simulink library "carnotUIBK"  (R2024b)
settings: Solver=VariableStepAuto  StartTime=0.0  StopTime=10.0  RelTol=1e-3  EnableMultiTasking=on
values from neighbouring files (symbols this model uses):
  area = area + room(kk).area    [THERMALZONE.m]
  boundary = BOUNDARY()    [BUILDING.m]
  building = obj    [BUILDING.m]
  C = zeros(1,length(d)+1)    [CONSTRUCTION.m]
  cp = str2num(value)    [CONSTRUCTION.m]
  pos = find(d_layer>0)    [CONSTRUCTION.m]
  rho = str2num(value)    [CONSTRUCTION.m]
  type = 1    [CONSTRUCTION.m]
  zone = obj.zone(ind)    [THERMALZONE.m]
undefined symbols (not defined in the file or in its folder): A, amb_factor, B, const, control, Dd, get_building, height, p, Qdot_C, Qdot_H, Qdot_I_electricity, Qdot_I_light, Qdot_I_person, Qdot_S, Qdot_T_ground, Qdot_T_neighbour, Qdot_T_opaque, Qdot_T_window, Qdot_V_infiltration, Qdot_V_mech, Qdot_V_window, r_frame, solar_ratio, solar_ratio1, solar_ratio2, Tc, Tr, Ts, Uvalue, view_factor, wall, wallsurface, window, window_height, window_heigth, window_width, windowsurface, x_CO2, x_H2O, x_VOC, z
libraries: carnot x105, $bdroot x22, simulink x18, simulink_extras x14
(part 6 of 13)

== system carnotUIBK/HVAC/HVAC_2001_ventilation system simple/ventilation_zone 6 ==
  note: ASSUMPTION: mdot_air_in = mdot_air_out !
  note: AIR VENTILATION outdoors - indoors
  note: x_sup = x_amb + (x_ext - x_amb) * eta_x
  AIB : Inport
  WDB : Inport  Port=2
  Vdot : Inport  Port=3
  Enable : EnablePort
  "\"air\"" : Constant  Value=2
  "1/h -> 1/s" : Gain  Gain=1/3600  SaturateOnIntegerOverflow=on  OutDataTypeStr=Inherit: Same as input  ParamDataTypeStr=Inherit: Same as input
  Bus Creator1 : BusCreator  Inputs=2
  Bus Selector : BusSelector  OutputSignals=Temperature_Ambient,Relative_Humidity,Station_Pressure
  Bus Selector1 : BusSelector  OutputSignals=Tc,x_H2O,x_CO2
  Constant : Constant  Value=zeros(1,2)
  Constant1 : Constant  Value=zeros(1,5)
  Constant2 : Constant  Value=zeros(1,7)
  Constant3 : Constant  Value=1-eta
  Constant4 : Constant  Value=0
  Constant5 : Constant  Value=eta_x
  Density : carnot/Basic/Material_Properties/Density  VariantControl=CarlibClassic  INPUTARGUMENTS=state variables (classic)  DEBUGLEVEL=NOLEVEL  MAXTOTALWARNINGS=inf  MAXCONSECUTIVEWARNINGS=inf  WRITETOFILE=0  FILENAME='errors.txt'
      settings: SourceProductName=Carnot
  Fcn : Fcn  Expr=u / (1+u)
  Fcn1 : Fcn  Expr=u / (1+u)
  Integrator : Integrator
  Mux1 : Mux  Inputs=[1 1]
  Mux3 : Mux  Inputs=[1 2 1 1 1 5 1 7]
  Mux4 : Mux  Inputs=2
  Product1 : Product  InputSameDT=on  SaturateOnIntegerOverflow=on  OutDataTypeStr=Inherit: Same as first input
  Product2 : Product  InputSameDT=on  SaturateOnIntegerOverflow=on  OutDataTypeStr=Inherit: Same as first input
  Product3 : Product  InputSameDT=on  SaturateOnIntegerOverflow=on  OutDataTypeStr=Inherit: Same as first input
  Product4 : Product  Inputs=4  InputSameDT=on  SaturateOnIntegerOverflow=on  OutDataTypeStr=Inherit: Same as first input
  RelHum2x : carnot/Basic/Material_Properties/RelHum2x
      settings: SourceProductName=Carnot
  Subsystem : Subsystem
  Sum : Sum  Inputs=-+  InputSameDT=on  SaturateOnIntegerOverflow=on  OutDataTypeStr=Inherit: Same as first input
  Sum1 : Sum  Inputs=-+  InputSameDT=on  SaturateOnIntegerOverflow=on  OutDataTypeStr=Inherit: Same as first input
  Sum2 : Sum  Inputs=++-  InputSameDT=on  SaturateOnIntegerOverflow=on  OutDataTypeStr=Inherit: Same as first input
  Terminator : Terminator
  cp Constant : Constant  Value=1006.8
  rho(CO2) / rho(air) * CO2norm (kg/kg) : Constant  Value=1.529*CO2norm
  "[S]" : Outport  VectorParamsAs1DForOutWhenUnconnected=off
  "[HVAC]" : Outport  Port=2  VectorParamsAs1DForOutWhenUnconnected=off
  wires:
  Fcn1/1 -> Sum2/1, Sum1/1
  Fcn/1 -> Sum1/2, Sum2/3
  Product2/1 -> Mux3/4  "mdot_H2O"
  Sum2/1 -> Product2/2  "x_sup"
  Product1/1 -> Sum2/2
  Sum1/1 -> Product1/2
  Constant5/1 -> Product1/1
  Subsystem/1(mdot_H2O) -> Terminator/1  "mdot_H2O"
  Constant4/1 -> Mux3/3
  Vdot/1 -> "1/h -> 1/s"/1
  Mux3/1 -> "[S]"/1
  Subsystem/2(mdot_CO2) -> Mux3/5  "mdot_CO2"
  WDB/1 -> Bus Selector/1
  AIB/1 -> Bus Selector1/1
  Density/1 -> Product3/2
  Bus Selector/3 -> RelHum2x/2, Density/2  "<Station_Pressure>"
  Bus Selector/2 -> RelHum2x/3  "<Relative_Humidity>"
  Bus Selector/1 -> RelHum2x/1, Density/1, Sum/2  "<Temperature_Ambient>"
  RelHum2x/1 -> Density/4, Mux4/1, Fcn1/1  "x_H2O"
  "\"air\""/1 -> Density/3
  Mux1/1 -> Subsystem/2(x_in)  "[x_H2O, x_CO2]_in"
  Bus Selector1/1 -> Sum/1  "<Tc>"
  Mux4/1 -> Subsystem/3(x_out)
  rho(CO2) / rho(air) * CO2norm (kg/kg)/1 -> Mux4/2  "x_CO2"
  Sum/1 -> Product4/2  "dT"
  cp Constant/1 -> Product4/3  "cp"
  Product3/1 -> Product4/4, Product2/1, Subsystem/1(mdot_air)
  Bus Selector1/2 -> Mux1/1, Fcn/1  "<x_H2O>"
  Bus Selector1/3 -> Mux1/2  "<x_CO2>"
  Constant/1 -> Mux3/2
  Constant1/1 -> Mux3/6
  Constant2/1 -> Mux3/8
  Constant3/1 -> Product4/1
  "1/h -> 1/s"/1 -> Product3/1
  Bus Creator1/1 -> "[HVAC]"/1
  Product4/1 -> Mux3/7, Integrator/1, Bus Creator1/1, Mux3/1  "ventilation power"
  Integrator/1 -> Bus Creator1/2  "ventilation energy"

== system carnotUIBK/HVAC/HVAC_2001_ventilation system simple/ventilation_zone 7 ==
  note: ASSUMPTION: mdot_air_in = mdot_air_out !
  note: AIR VENTILATION outdoors - indoors
  note: x_sup = x_amb + (x_ext - x_amb) * eta_x
  AIB : Inport
  WDB : Inport  Port=2
  Vdot : Inport  Port=3
  Enable : EnablePort
  "\"air\"" : Constant  Value=2
  "1/h -> 1/s" : Gain  Gain=1/3600  SaturateOnIntegerOverflow=on  OutDataTypeStr=Inherit: Same as input  ParamDataTypeStr=Inherit: Same as input
  Bus Creator1 : BusCreator  Inputs=2
  Bus Selector : BusSelector  OutputSignals=Temperature_Ambient,Relative_Humidity,Station_Pressure
  Bus Selector1 : BusSelector  OutputSignals=Tc,x_H2O,x_CO2
  Constant : Constant  Value=zeros(1,2)
  Constant1 : Constant  Value=zeros(1,5)
  Constant2 : Constant  Value=zeros(1,7)
  Constant3 : Constant  Value=1-eta
  Constant4 : Constant  Value=0
  Constant5 : Constant  Value=eta_x
  Density : carnot/Basic/Material_Properties/Density  VariantControl=CarlibClassic  INPUTARGUMENTS=state variables (classic)  DEBUGLEVEL=NOLEVEL  MAXTOTALWARNINGS=inf  MAXCONSECUTIVEWARNINGS=inf  WRITETOFILE=0  FILENAME='errors.txt'
      settings: SourceProductName=Carnot
  Fcn : Fcn  Expr=u / (1+u)
  Fcn1 : Fcn  Expr=u / (1+u)
  Integrator : Integrator
  Mux1 : Mux  Inputs=[1 1]
  Mux3 : Mux  Inputs=[1 2 1 1 1 5 1 7]
  Mux4 : Mux  Inputs=2
  Product1 : Product  InputSameDT=on  SaturateOnIntegerOverflow=on  OutDataTypeStr=Inherit: Same as first input
  Product2 : Product  InputSameDT=on  SaturateOnIntegerOverflow=on  OutDataTypeStr=Inherit: Same as first input
  Product3 : Product  InputSameDT=on  SaturateOnIntegerOverflow=on  OutDataTypeStr=Inherit: Same as first input
  Product4 : Product  Inputs=4  InputSameDT=on  SaturateOnIntegerOverflow=on  OutDataTypeStr=Inherit: Same as first input
  RelHum2x : carnot/Basic/Material_Properties/RelHum2x
      settings: SourceProductName=Carnot
  Subsystem : Subsystem
  Sum : Sum  Inputs=-+  InputSameDT=on  SaturateOnIntegerOverflow=on  OutDataTypeStr=Inherit: Same as first input
  Sum1 : Sum  Inputs=-+  InputSameDT=on  SaturateOnIntegerOverflow=on  OutDataTypeStr=Inherit: Same as first input
  Sum2 : Sum  Inputs=++-  InputSameDT=on  SaturateOnIntegerOverflow=on  OutDataTypeStr=Inherit: Same as first input
  Terminator : Terminator
  cp Constant : Constant  Value=1006.8
  rho(CO2) / rho(air) * CO2norm (kg/kg) : Constant  Value=1.529*CO2norm
  "[S]" : Outport  VectorParamsAs1DForOutWhenUnconnected=off
  "[HVAC]" : Outport  Port=2  VectorParamsAs1DForOutWhenUnconnected=off
  wires:
  Fcn1/1 -> Sum2/1, Sum1/1
  Fcn/1 -> Sum1/2, Sum2/3
  Product2/1 -> Mux3/4  "mdot_H2O"
  Sum2/1 -> Product2/2  "x_sup"
  Product1/1 -> Sum2/2
  Sum1/1 -> Product1/2
  Constant5/1 -> Product1/1
  Subsystem/1(mdot_H2O) -> Terminator/1  "mdot_H2O"
  Constant4/1 -> Mux3/3
  Vdot/1 -> "1/h -> 1/s"/1
  Mux3/1 -> "[S]"/1
  Subsystem/2(mdot_CO2) -> Mux3/5  "mdot_CO2"
  WDB/1 -> Bus Selector/1
  AIB/1 -> Bus Selector1/1
  Density/1 -> Product3/2
  Bus Selector/3 -> RelHum2x/2, Density/2  "<Station_Pressure>"
  Bus Selector/2 -> RelHum2x/3  "<Relative_Humidity>"
  Bus Selector/1 -> RelHum2x/1, Density/1, Sum/2  "<Temperature_Ambient>"
  RelHum2x/1 -> Density/4, Mux4/1, Fcn1/1  "x_H2O"
  "\"air\""/1 -> Density/3
  Mux1/1 -> Subsystem/2(x_in)  "[x_H2O, x_CO2]_in"
  Bus Selector1/1 -> Sum/1  "<Tc>"
  Mux4/1 -> Subsystem/3(x_out)
  rho(CO2) / rho(air) * CO2norm (kg/kg)/1 -> Mux4/2  "x_CO2"
  Sum/1 -> Product4/2  "dT"
  cp Constant/1 -> Product4/3  "cp"
  Product3/1 -> Product4/4, Product2/1, Subsystem/1(mdot_air)
  Bus Selector1/2 -> Mux1/1, Fcn/1  "<x_H2O>"
  Bus Selector1/3 -> Mux1/2  "<x_CO2>"
  Constant/1 -> Mux3/2
  Constant1/1 -> Mux3/6
  Constant2/1 -> Mux3/8
  Constant3/1 -> Product4/1
  "1/h -> 1/s"/1 -> Product3/1
  Bus Creator1/1 -> "[HVAC]"/1
  Product4/1 -> Mux3/7, Integrator/1, Bus Creator1/1, Mux3/1  "ventilation power"
  Integrator/1 -> Bus Creator1/2  "ventilation energy"

== system carnotUIBK/HVAC/HVAC_2001_ventilation system simple/ventilation_zone 8 ==
  note: ASSUMPTION: mdot_air_in = mdot_air_out !
  note: AIR VENTILATION outdoors - indoors
  note: x_sup = x_amb + (x_ext - x_amb) * eta_x
  AIB : Inport
  WDB : Inport  Port=2
  Vdot : Inport  Port=3
  Enable : EnablePort
  "\"air\"" : Constant  Value=2
  "1/h -> 1/s" : Gain  Gain=1/3600  SaturateOnIntegerOverflow=on  OutDataTypeStr=Inherit: Same as input  ParamDataTypeStr=Inherit: Same as input
  Bus Creator1 : BusCreator  Inputs=2
  Bus Selector : BusSelector  OutputSignals=Temperature_Ambient,Relative_Humidity,Station_Pressure
  Bus Selector1 : BusSelector  OutputSignals=Tc,x_H2O,x_CO2
  Constant : Constant  Value=zeros(1,2)
  Constant1 : Constant  Value=zeros(1,5)
  Constant2 : Constant  Value=zeros(1,7)
  Constant3 : Constant  Value=1-eta
  Constant4 : Constant  Value=0
  Constant5 : Constant  Value=eta_x
  Density : carnot/Basic/Material_Properties/Density  VariantControl=CarlibClassic  INPUTARGUMENTS=state variables (classic)  DEBUGLEVEL=NOLEVEL  MAXTOTALWARNINGS=inf  MAXCONSECUTIVEWARNINGS=inf  WRITETOFILE=0  FILENAME='errors.txt'
      settings: SourceProductName=Carnot
  Fcn : Fcn  Expr=u / (1+u)
  Fcn1 : Fcn  Expr=u / (1+u)
  Integrator : Integrator
  Mux1 : Mux  Inputs=[1 1]
  Mux3 : Mux  Inputs=[1 2 1 1 1 5 1 7]
  Mux4 : Mux  Inputs=2
  Product1 : Product  InputSameDT=on  SaturateOnIntegerOverflow=on  OutDataTypeStr=Inherit: Same as first input
  Product2 : Product  InputSameDT=on  SaturateOnIntegerOverflow=on  OutDataTypeStr=Inherit: Same as first input
  Product3 : Product  InputSameDT=on  SaturateOnIntegerOverflow=on  OutDataTypeStr=Inherit: Same as first input
  Product4 : Product  Inputs=4  InputSameDT=on  SaturateOnIntegerOverflow=on  OutDataTypeStr=Inherit: Same as first input
  RelHum2x : carnot/Basic/Material_Properties/RelHum2x
      settings: SourceProductName=Carnot
  Subsystem : Subsystem
  Sum : Sum  Inputs=-+  InputSameDT=on  SaturateOnIntegerOverflow=on  OutDataTypeStr=Inherit: Same as first input
  Sum1 : Sum  Inputs=-+  InputSameDT=on  SaturateOnIntegerOverflow=on  OutDataTypeStr=Inherit: Same as first input
  Sum2 : Sum  Inputs=++-  InputSameDT=on  SaturateOnIntegerOverflow=on  OutDataTypeStr=Inherit: Same as first input
  Terminator : Terminator
  cp Constant : Constant  Value=1006.8
  rho(CO2) / rho(air) * CO2norm (kg/kg) : Constant  Value=1.529*CO2norm
  "[S]" : Outport  VectorParamsAs1DForOutWhenUnconnected=off
  "[HVAC]" : Outport  Port=2  VectorParamsAs1DForOutWhenUnconnected=off
  wires:
  Fcn1/1 -> Sum2/1, Sum1/1
  Fcn/1 -> Sum1/2, Sum2/3
  Product2/1 -> Mux3/4  "mdot_H2O"
  Sum2/1 -> Product2/2  "x_sup"
  Product1/1 -> Sum2/2
  Sum1/1 -> Product1/2
  Constant5/1 -> Product1/1
  Subsystem/1(mdot_H2O) -> Terminator/1  "mdot_H2O"
  Constant4/1 -> Mux3/3
  Vdot/1 -> "1/h -> 1/s"/1
  Mux3/1 -> "[S]"/1
  Subsystem/2(mdot_CO2) -> Mux3/5  "mdot_CO2"
  WDB/1 -> Bus Selector/1
  AIB/1 -> Bus Selector1/1
  Density/1 -> Product3/2
  Bus Selector/3 -> RelHum2x/2, Density/2  "<Station_Pressure>"
  Bus Selector/2 -> RelHum2x/3  "<Relative_Humidity>"
  Bus Selector/1 -> RelHum2x/1, Density/1, Sum/2  "<Temperature_Ambient>"
  RelHum2x/1 -> Density/4, Mux4/1, Fcn1/1  "x_H2O"
  "\"air\""/1 -> Density/3
  Mux1/1 -> Subsystem/2(x_in)  "[x_H2O, x_CO2]_in"
  Bus Selector1/1 -> Sum/1  "<Tc>"
  Mux4/1 -> Subsystem/3(x_out)
  rho(CO2) / rho(air) * CO2norm (kg/kg)/1 -> Mux4/2  "x_CO2"
  Sum/1 -> Product4/2  "dT"
  cp Constant/1 -> Product4/3  "cp"
  Product3/1 -> Product4/4, Product2/1, Subsystem/1(mdot_air)
  Bus Selector1/2 -> Mux1/1, Fcn/1  "<x_H2O>"
  Bus Selector1/3 -> Mux1/2  "<x_CO2>"
  Constant/1 -> Mux3/2
  Constant1/1 -> Mux3/6
  Constant2/1 -> Mux3/8
  Constant3/1 -> Product4/1
  "1/h -> 1/s"/1 -> Product3/1
  Bus Creator1/1 -> "[HVAC]"/1
  Product4/1 -> Mux3/7, Integrator/1, Bus Creator1/1, Mux3/1  "ventilation power"
  Integrator/1 -> Bus Creator1/2  "ventilation energy"

== system carnotUIBK/HVAC/HVAC_2001_ventilation system simple/ventilation_zone 9 ==
  note: ASSUMPTION: mdot_air_in = mdot_air_out !
  note: AIR VENTILATION outdoors - indoors
  note: x_sup = x_amb + (x_ext - x_amb) * eta_x
  AIB : Inport
  WDB : Inport  Port=2
  Vdot : Inport  Port=3
  Enable : EnablePort
  "\"air\"" : Constant  Value=2
  "1/h -> 1/s" : Gain  Gain=1/3600  SaturateOnIntegerOverflow=on  OutDataTypeStr=Inherit: Same as input  ParamDataTypeStr=Inherit: Same as input
  Bus Creator1 : BusCreator  Inputs=2
  Bus Selector : BusSelector  OutputSignals=Temperature_Ambient,Relative_Humidity,Station_Pressure
  Bus Selector1 : BusSelector  OutputSignals=Tc,x_H2O,x_CO2
  Constant : Constant  Value=zeros(1,2)
  Constant1 : Constant  Value=zeros(1,5)
  Constant2 : Constant  Value=zeros(1,7)
  Constant3 : Constant  Value=1-eta
  Constant4 : Constant  Value=0
  Constant5 : Constant  Value=eta_x
  Density : carnot/Basic/Material_Properties/Density  VariantControl=CarlibClassic  INPUTARGUMENTS=state variables (classic)  DEBUGLEVEL=NOLEVEL  MAXTOTALWARNINGS=inf  MAXCONSECUTIVEWARNINGS=inf  WRITETOFILE=0  FILENAME='errors.txt'
      settings: SourceProductName=Carnot
  Fcn : Fcn  Expr=u / (1+u)
  Fcn1 : Fcn  Expr=u / (1+u)
  Integrator : Integrator
  Mux1 : Mux  Inputs=[1 1]
  Mux3 : Mux  Inputs=[1 2 1 1 1 5 1 7]
  Mux4 : Mux  Inputs=2
  Product1 : Product  InputSameDT=on  SaturateOnIntegerOverflow=on  OutDataTypeStr=Inherit: Same as first input
  Product2 : Product  InputSameDT=on  SaturateOnIntegerOverflow=on  OutDataTypeStr=Inherit: Same as first input
  Product3 : Product  InputSameDT=on  SaturateOnIntegerOverflow=on  OutDataTypeStr=Inherit: Same as first input
  Product4 : Product  Inputs=4  InputSameDT=on  SaturateOnIntegerOverflow=on  OutDataTypeStr=Inherit: Same as first input
  RelHum2x : carnot/Basic/Material_Properties/RelHum2x
      settings: SourceProductName=Carnot
  Subsystem : Subsystem
  Sum : Sum  Inputs=-+  InputSameDT=on  SaturateOnIntegerOverflow=on  OutDataTypeStr=Inherit: Same as first input
  Sum1 : Sum  Inputs=-+  InputSameDT=on  SaturateOnIntegerOverflow=on  OutDataTypeStr=Inherit: Same as first input
  Sum2 : Sum  Inputs=++-  InputSameDT=on  SaturateOnIntegerOverflow=on  OutDataTypeStr=Inherit: Same as first input
  Terminator : Terminator
  cp Constant : Constant  Value=1006.8
  rho(CO2) / rho(air) * CO2norm (kg/kg) : Constant  Value=1.529*CO2norm
  "[S]" : Outport  VectorParamsAs1DForOutWhenUnconnected=off
  "[HVAC]" : Outport  Port=2  VectorParamsAs1DForOutWhenUnconnected=off
  wires:
  Fcn1/1 -> Sum2/1, Sum1/1
  Fcn/1 -> Sum1/2, Sum2/3
  Product2/1 -> Mux3/4  "mdot_H2O"
  Sum2/1 -> Product2/2  "x_sup"
  Product1/1 -> Sum2/2
  Sum1/1 -> Product1/2
  Constant5/1 -> Product1/1
  Subsystem/1(mdot_H2O) -> Terminator/1  "mdot_H2O"
  Constant4/1 -> Mux3/3
  Vdot/1 -> "1/h -> 1/s"/1
  Mux3/1 -> "[S]"/1
  Subsystem/2(mdot_CO2) -> Mux3/5  "mdot_CO2"
  WDB/1 -> Bus Selector/1
  AIB/1 -> Bus Selector1/1
  Density/1 -> Product3/2
  Bus Selector/3 -> RelHum2x/2, Density/2  "<Station_Pressure>"
  Bus Selector/2 -> RelHum2x/3  "<Relative_Humidity>"
  Bus Selector/1 -> RelHum2x/1, Density/1, Sum/2  "<Temperature_Ambient>"
  RelHum2x/1 -> Density/4, Mux4/1, Fcn1/1  "x_H2O"
  "\"air\""/1 -> Density/3
  Mux1/1 -> Subsystem/2(x_in)  "[x_H2O, x_CO2]_in"
  Bus Selector1/1 -> Sum/1  "<Tc>"
  Mux4/1 -> Subsystem/3(x_out)
  rho(CO2) / rho(air) * CO2norm (kg/kg)/1 -> Mux4/2  "x_CO2"
  Sum/1 -> Product4/2  "dT"
  cp Constant/1 -> Product4/3  "cp"
  Product3/1 -> Product4/4, Product2/1, Subsystem/1(mdot_air)
  Bus Selector1/2 -> Mux1/1, Fcn/1  "<x_H2O>"
  Bus Selector1/3 -> Mux1/2  "<x_CO2>"
  Constant/1 -> Mux3/2
  Constant1/1 -> Mux3/6
  Constant2/1 -> Mux3/8
  Constant3/1 -> Product4/1
  "1/h -> 1/s"/1 -> Product3/1
  Bus Creator1/1 -> "[HVAC]"/1
  Product4/1 -> Mux3/7, Integrator/1, Bus Creator1/1, Mux3/1  "ventilation power"
  Integrator/1 -> Bus Creator1/2  "ventilation energy"

== system carnotUIBK/HVAC/HVAC_9001_window shading/Transfer Fcn (with initial states) ==
  In1 : Inport
  State Space : StateSpace  A=A  B=B  C=C  D=Dd  InitialCondition=X0
  Out1 : Outport  InitialOutput=0  VectorParamsAs1DForOutWhenUnconnected=off
  wires:
  In1/1 -> State Space/1
  State Space/1 -> Out1/1

== system carnotUIBK/HVAC/HVAC_9002_window opening/window opening 1 ==
  setpoint : Inport
  AIB : Inport  Port=2
  WDB : Inport  Port=3
  Enable : EnablePort
  Add : Sum
  Bus Selector1 : BusSelector  OutputSignals=Temperature_Ambient
  Bus Selector5 : BusSelector  OutputSignals=Ts,Tc,p,x_H2O
  Product : Product
  Saturation : Saturate  UpperLimit=1  LowerLimit=0
  Sum : Sum  Inputs=|-+
  Sum1 : Sum  Inputs=|+-
  Sum2 : Sum  Inputs=|-+
  Transfer Fcn (with initial states) : Subsystem  mask(Transfer Function with Initial States){N=[1], D=[600 1], X0=0}
      mask prompts: N "Numerator:"; D "Denominator:"; X0 "Initial conditions:"
      mask help: Vector expressions for numerator, and denominator. Coefficients are in descending powers of s.
      mask init:
      | [A,B,C,Dd]=tf2ss(N,D);if (isempty(X0));[m,n]=size(A);X0=zeros(1,m); end;
      mask Help: Specify the initial states for the transfer function.  The state ordering is determined by the m-file tf2ss.  There is no unique mapping of the states in a transfer function to states in a state-space representation.  However, tf2ss will consistently use the same mapping for a given transfer function.
      mask Display: dpoly(N,D,'s')
  Transfer Fcn (with initial states)1 : Subsystem  mask(Transfer Function with Initial States){N=[1], D=[600 1], X0=0}
      mask prompts: N "Numerator:"; D "Denominator:"; X0 "Initial conditions:"
      mask help: Vector expressions for numerator, and denominator. Coefficients are in descending powers of s.
      mask init:
      | [A,B,C,Dd]=tf2ss(N,D);if (isempty(X0));[m,n]=size(A);X0=zeros(1,m); end;
      mask Help: Specify the initial states for the transfer function.  The state ordering is determined by the m-file tf2ss.  There is no unique mapping of the states in a transfer function to states in a state-space representation.  However, tf2ss will consistently use the same mapping for a given transfer function.
      mask Display: dpoly(N,D,'s')
  Transfer Fcn (with initial states)2 : Subsystem  mask(Transfer Function with Initial States){N=[1], D=[600 1], X0=0}
      mask prompts: N "Numerator:"; D "Denominator:"; X0 "Initial conditions:"
      mask help: Vector expressions for numerator, and denominator. Coefficients are in descending powers of s.
      mask init:
      | [A,B,C,Dd]=tf2ss(N,D);if (isempty(X0));[m,n]=size(A);X0=zeros(1,m); end;
      mask Help: Specify the initial states for the transfer function.  The state ordering is determined by the m-file tf2ss.  There is no unique mapping of the states in a transfer function to states in a state-space representation.  However, tf2ss will consistently use the same mapping for a given transfer function.
      mask Display: dpoly(N,D,'s')
  on/off ambient : Relay  OnSwitchValue=0.5  OffSwitchValue=-0.5
  on/off hum : Relay  OnSwitchValue=0.5  OffSwitchValue=-0.5
  on/off roomtemp : Relay  OnSwitchValue=0.5  OffSwitchValue=-0.5
  setpoint humidity : Constant  Value=85
  x2RelHum_UIBK : carnot/Basic/Material_Properties/x2RelHum
      settings: SourceProductName=Carnot
  state : Outport  VectorParamsAs1DForOutWhenUnconnected=off
  wires:
  AIB/1 -> Bus Selector5/1
  setpoint/1 -> Sum/1
  Bus Selector5/1 -> Transfer Fcn (with initial states)/1(In1)  "<Ts>"
  Sum/1 -> on/off roomtemp/1
  on/off roomtemp/1 -> Product/1
  WDB/1 -> Bus Selector1/1
  Bus Selector1/1 -> Transfer Fcn (with initial states)2/1(In1)  "<Temperature_Ambient>"
  Sum1/1 -> on/off ambient/1
  on/off ambient/1 -> Product/2
  Bus Selector5/2 -> x2RelHum_UIBK/1  "<Tc>"
  Bus Selector5/3 -> x2RelHum_UIBK/2  "<p>"
  Bus Selector5/4 -> x2RelHum_UIBK/3  "<x_H2O>"
  Sum2/1 -> on/off hum/1
  x2RelHum_UIBK/1 -> Transfer Fcn (with initial states)1/1(In1)
  setpoint humidity/1 -> Sum2/1
  Add/1 -> Saturation/1
  Product/1 -> Add/2
  on/off hum/1 -> Add/1
  Saturation/1 -> state/1
  Transfer Fcn (with initial states)/1(Out1) -> Sum1/1, Sum/2
  Transfer Fcn (with initial states)2/1(Out1) -> Sum1/2
  Transfer Fcn (with initial states)1/1(Out1) -> Sum2/2

== system carnotUIBK/HVAC/HVAC_9002_window opening/window opening 2 ==
  setpoint : Inport
  AIB : Inport  Port=2
  WDB : Inport  Port=3
  Enable : EnablePort
  Add : Sum
  Bus Selector1 : BusSelector  OutputSignals=Temperature_Ambient
  Bus Selector5 : BusSelector  OutputSignals=Ts,Tc,p,x_H2O
  Product : Product
  Saturation : Saturate  UpperLimit=1  LowerLimit=0
  Sum : Sum  Inputs=|-+
  Sum1 : Sum  Inputs=|+-
  Sum2 : Sum  Inputs=|-+
  Transfer Fcn (with initial states)1 : Subsystem  mask(Transfer Function with Initial States){N=[1], D=[600 1], X0=0}
      mask prompts: N "Numerator:"; D "Denominator:"; X0 "Initial conditions:"
      mask help: Vector expressions for numerator, and denominator. Coefficients are in descending powers of s.
      mask init:
      | [A,B,C,Dd]=tf2ss(N,D);if (isempty(X0));[m,n]=size(A);X0=zeros(1,m); end;
      mask Help: Specify the initial states for the transfer function.  The state ordering is determined by the m-file tf2ss.  There is no unique mapping of the states in a transfer function to states in a state-space representation.  However, tf2ss will consistently use the same mapping for a given transfer function.
      mask Display: dpoly(N,D,'s')
  Transfer Fcn (with initial states)2 : Subsystem  mask(Transfer Function with Initial States){N=[1], D=[600 1], X0=0}
      mask prompts: N "Numerator:"; D "Denominator:"; X0 "Initial conditions:"
      mask help: Vector expressions for numerator, and denominator. Coefficients are in descending powers of s.
      mask init:
      | [A,B,C,Dd]=tf2ss(N,D);if (isempty(X0));[m,n]=size(A);X0=zeros(1,m); end;
      mask Help: Specify the initial states for the transfer function.  The state ordering is determined by the m-file tf2ss.  There is no unique mapping of the states in a transfer function to states in a state-space representation.  However, tf2ss will consistently use the same mapping for a given transfer function.
      mask Display: dpoly(N,D,'s')
  Transfer Fcn (with initial states)3 : Subsystem  mask(Transfer Function with Initial States){N=[1], D=[600 1], X0=0}
      mask prompts: N "Numerator:"; D "Denominator:"; X0 "Initial conditions:"
      mask help: Vector expressions for numerator, and denominator. Coefficients are in descending powers of s.
      mask init:
      | [A,B,C,Dd]=tf2ss(N,D);if (isempty(X0));[m,n]=size(A);X0=zeros(1,m); end;
      mask Help: Specify the initial states for the transfer function.  The state ordering is determined by the m-file tf2ss.  There is no unique mapping of the states in a transfer function to states in a state-space representation.  However, tf2ss will consistently use the same mapping for a given transfer function.
      mask Display: dpoly(N,D,'s')
  on/off ambient : Relay  OnSwitchValue=0.5  OffSwitchValue=-0.5
  on/off hum : Relay  OnSwitchValue=0.5  OffSwitchValue=-0.5
  on/off roomtemp : Relay  OnSwitchValue=0.5  OffSwitchValue=-0.5
  setpoint humidity : Constant  Value=85
  x2RelHum_UIBK : carnot/Basic/Material_Properties/x2RelHum
      settings: SourceProductName=Carnot
  state : Outport  VectorParamsAs1DForOutWhenUnconnected=off
  wires:
  Transfer Fcn (with initial states)1/1(Out1) -> Sum2/2
  Transfer Fcn (with initial states)3/1(Out1) -> Sum1/2
  Transfer Fcn (with initial states)2/1(Out1) -> Sum/2, Sum1/1
  Saturation/1 -> state/1
  on/off hum/1 -> Add/1
  Product/1 -> Add/2
  Add/1 -> Saturation/1
  setpoint humidity/1 -> Sum2/1
  x2RelHum_UIBK/1 -> Transfer Fcn (with initial states)1/1(In1)
  Sum2/1 -> on/off hum/1
  Bus Selector5/4 -> x2RelHum_UIBK/3  "<x_H2O>"
  Bus Selector5/3 -> x2RelHum_UIBK/2  "<p>"
  Bus Selector5/2 -> x2RelHum_UIBK/1  "<Tc>"
  on/off ambient/1 -> Product/2
  Sum1/1 -> on/off ambient/1
  Bus Selector1/1 -> Transfer Fcn (with initial states)3/1(In1)  "<Temperature_Ambient>"
  WDB/1 -> Bus Selector1/1
  on/off roomtemp/1 -> Product/1
  Sum/1 -> on/off roomtemp/1
  Bus Selector5/1 -> Transfer Fcn (with initial states)2/1(In1)  "<Ts>"
  setpoint/1 -> Sum/1
  AIB/1 -> Bus Selector5/1

== system carnotUIBK/HVAC/HVAC_9002_window opening/window opening 3 ==
  setpoint : Inport
  AIB : Inport  Port=2
  WDB : Inport  Port=3
  Enable : EnablePort
  Add : Sum
  Bus Selector1 : BusSelector  OutputSignals=Temperature_Ambient
  Bus Selector5 : BusSelector  OutputSignals=Ts,Tc,p,x_H2O
  Product : Product
  Saturation : Saturate  UpperLimit=1  LowerLimit=0
  Sum : Sum  Inputs=|-+
  Sum1 : Sum  Inputs=|+-
  Sum2 : Sum  Inputs=|-+
  Transfer Fcn (with initial states)1 : Subsystem  mask(Transfer Function with Initial States){N=[1], D=[600 1], X0=0}
      mask prompts: N "Numerator:"; D "Denominator:"; X0 "Initial conditions:"
      mask help: Vector expressions for numerator, and denominator. Coefficients are in descending powers of s.
      mask init:
      | [A,B,C,Dd]=tf2ss(N,D);if (isempty(X0));[m,n]=size(A);X0=zeros(1,m); end;
      mask Help: Specify the initial states for the transfer function.  The state ordering is determined by the m-file tf2ss.  There is no unique mapping of the states in a transfer function to states in a state-space representation.  However, tf2ss will consistently use the same mapping for a given transfer function.
      mask Display: dpoly(N,D,'s')
  Transfer Fcn (with initial states)2 : Subsystem  mask(Transfer Function with Initial States){N=[1], D=[600 1], X0=0}
      mask prompts: N "Numerator:"; D "Denominator:"; X0 "Initial conditions:"
      mask help: Vector expressions for numerator, and denominator. Coefficients are in descending powers of s.
      mask init:
      | [A,B,C,Dd]=tf2ss(N,D);if (isempty(X0));[m,n]=size(A);X0=zeros(1,m); end;
      mask Help: Specify the initial states for the transfer function.  The state ordering is determined by the m-file tf2ss.  There is no unique mapping of the states in a transfer function to states in a state-space representation.  However, tf2ss will consistently use the same mapping for a given transfer function.
      mask Display: dpoly(N,D,'s')
  Transfer Fcn (with initial states)3 : Subsystem  mask(Transfer Function with Initial States){N=[1], D=[600 1], X0=0}
      mask prompts: N "Numerator:"; D "Denominator:"; X0 "Initial conditions:"
      mask help: Vector expressions for numerator, and denominator. Coefficients are in descending powers of s.
      mask init:
      | [A,B,C,Dd]=tf2ss(N,D);if (isempty(X0));[m,n]=size(A);X0=zeros(1,m); end;
      mask Help: Specify the initial states for the transfer function.  The state ordering is determined by the m-file tf2ss.  There is no unique mapping of the states in a transfer function to states in a state-space representation.  However, tf2ss will consistently use the same mapping for a given transfer function.
      mask Display: dpoly(N,D,'s')
  on/off ambient : Relay  OnSwitchValue=0.5  OffSwitchValue=-0.5
  on/off hum : Relay  OnSwitchValue=0.5  OffSwitchValue=-0.5
  on/off roomtemp : Relay  OnSwitchValue=0.5  OffSwitchValue=-0.5
  setpoint humidity : Constant  Value=85
  x2RelHum_UIBK : carnot/Basic/Material_Properties/x2RelHum
      settings: SourceProductName=Carnot
  state : Outport  VectorParamsAs1DForOutWhenUnconnected=off
  wires:
  AIB/1 -> Bus Selector5/1
  setpoint/1 -> Sum/1
  Bus Selector5/1 -> Transfer Fcn (with initial states)3/1(In1)  "<Ts>"
  Sum/1 -> on/off roomtemp/1
  on/off roomtemp/1 -> Product/1
  WDB/1 -> Bus Selector1/1
  Bus Selector1/1 -> Transfer Fcn (with initial states)2/1(In1)  "<Temperature_Ambient>"
  Sum1/1 -> on/off ambient/1
  on/off ambient/1 -> Product/2
  Bus Selector5/2 -> x2RelHum_UIBK/1  "<Tc>"
  Bus Selector5/3 -> x2RelHum_UIBK/2  "<p>"
  Bus Selector5/4 -> x2RelHum_UIBK/3  "<x_H2O>"
  Sum2/1 -> on/off hum/1
  x2RelHum_UIBK/1 -> Transfer Fcn (with initial states)1/1(In1)
  setpoint humidity/1 -> Sum2/1
  Add/1 -> Saturation/1
  Product/1 -> Add/2
  on/off hum/1 -> Add/1
  Saturation/1 -> state/1
  Transfer Fcn (with initial states)3/1(Out1) -> Sum1/1, Sum/2
  Transfer Fcn (with initial states)2/1(Out1) -> Sum1/2
  Transfer Fcn (with initial states)1/1(Out1) -> Sum2/2

== system carnotUIBK/HVAC/HVAC_9002_window opening/window opening 4 ==
  setpoint : Inport
  AIB : Inport  Port=2
  WDB : Inport  Port=3
  Enable : EnablePort
  Add : Sum
  Bus Selector1 : BusSelector  OutputSignals=Temperature_Ambient
  Bus Selector5 : BusSelector  OutputSignals=Ts,Tc,p,x_H2O
  Product : Product
  Saturation : Saturate  UpperLimit=1  LowerLimit=0
  Sum : Sum  Inputs=|-+
  Sum1 : Sum  Inputs=|+-
  Sum2 : Sum  Inputs=|-+
  Transfer Fcn (with initial states)1 : Subsystem  mask(Transfer Function with Initial States){N=[1], D=[600 1], X0=0}
      mask prompts: N "Numerator:"; D "Denominator:"; X0 "Initial conditions:"
      mask help: Vector expressions for numerator, and denominator. Coefficients are in descending powers of s.
      mask init:
      | [A,B,C,Dd]=tf2ss(N,D);if (isempty(X0));[m,n]=size(A);X0=zeros(1,m); end;
      mask Help: Specify the initial states for the transfer function.  The state ordering is determined by the m-file tf2ss.  There is no unique mapping of the states in a transfer function to states in a state-space representation.  However, tf2ss will consistently use the same mapping for a given transfer function.
      mask Display: dpoly(N,D,'s')
  Transfer Fcn (with initial states)2 : Subsystem  mask(Transfer Function with Initial States){N=[1], D=[600 1], X0=0}
      mask prompts: N "Numerator:"; D "Denominator:"; X0 "Initial conditions:"
      mask help: Vector expressions for numerator, and denominator. Coefficients are in descending powers of s.
      mask init:
      | [A,B,C,Dd]=tf2ss(N,D);if (isempty(X0));[m,n]=size(A);X0=zeros(1,m); end;
      mask Help: Specify the initial states for the transfer function.  The state ordering is determined by the m-file tf2ss.  There is no unique mapping of the states in a transfer function to states in a state-space representation.  However, tf2ss will consistently use the same mapping for a given transfer function.
      mask Display: dpoly(N,D,'s')
  Transfer Fcn (with initial states)3 : Subsystem  mask(Transfer Function with Initial States){N=[1], D=[600 1], X0=0}
      mask prompts: N "Numerator:"; D "Denominator:"; X0 "Initial conditions:"
      mask help: Vector expressions for numerator, and denominator. Coefficients are in descending powers of s.
      mask init:
      | [A,B,C,Dd]=tf2ss(N,D);if (isempty(X0));[m,n]=size(A);X0=zeros(1,m); end;
      mask Help: Specify the initial states for the transfer function.  The state ordering is determined by the m-file tf2ss.  There is no unique mapping of the states in a transfer function to states in a state-space representation.  However, tf2ss will consistently use the same mapping for a given transfer function.
      mask Display: dpoly(N,D,'s')
  on/off ambient : Relay  OnSwitchValue=0.5  OffSwitchValue=-0.5
  on/off hum : Relay  OnSwitchValue=0.5  OffSwitchValue=-0.5
  on/off roomtemp : Relay  OnSwitchValue=0.5  OffSwitchValue=-0.5
  setpoint humidity : Constant  Value=85
  x2RelHum_UIBK : carnot/Basic/Material_Properties/x2RelHum
      settings: SourceProductName=Carnot
  state : Outport  VectorParamsAs1DForOutWhenUnconnected=off
  wires:
  Transfer Fcn (with initial states)1/1(Out1) -> Sum2/2
  Transfer Fcn (with initial states)2/1(Out1) -> Sum1/2
  Transfer Fcn (with initial states)3/1(Out1) -> Sum/2, Sum1/1
  Saturation/1 -> state/1
  on/off hum/1 -> Add/1
  Product/1 -> Add/2
  Add/1 -> Saturation/1
  setpoint humidity/1 -> Sum2/1
  x2RelHum_UIBK/1 -> Transfer Fcn (with initial states)1/1(In1)
  Sum2/1 -> on/off hum/1
  Bus Selector5/4 -> x2RelHum_UIBK/3  "<x_H2O>"
  Bus Selector5/3 -> x2RelHum_UIBK/2  "<p>"
  Bus Selector5/2 -> x2RelHum_UIBK/1  "<Tc>"
  on/off ambient/1 -> Product/2
  Sum1/1 -> on/off ambient/1
  Bus Selector1/1 -> Transfer Fcn (with initial states)2/1(In1)  "<Temperature_Ambient>"
  WDB/1 -> Bus Selector1/1
  on/off roomtemp/1 -> Product/1
  Sum/1 -> on/off roomtemp/1
  Bus Selector5/1 -> Transfer Fcn (with initial states)3/1(In1)  "<Ts>"
  setpoint/1 -> Sum/1
  AIB/1 -> Bus Selector5/1

== system carnotUIBK/HVAC/HVAC_9002_window opening/window opening 5 ==
  setpoint : Inport
  AIB : Inport  Port=2
  WDB : Inport  Port=3
  Enable : EnablePort
  Add : Sum
  Bus Selector1 : BusSelector  OutputSignals=Temperature_Ambient
  Bus Selector5 : BusSelector  OutputSignals=Ts,Tc,p,x_H2O
  Product : Product
  Saturation : Saturate  UpperLimit=1  LowerLimit=0
  Sum : Sum  Inputs=|-+
  Sum1 : Sum  Inputs=|+-
  Sum2 : Sum  Inputs=|-+
  Transfer Fcn (with initial states)1 : Subsystem  mask(Transfer Function with Initial States){N=[1], D=[600 1], X0=0}
      mask prompts: N "Numerator:"; D "Denominator:"; X0 "Initial conditions:"
      mask help: Vector expressions for numerator, and denominator. Coefficients are in descending powers of s.
      mask init:
      | [A,B,C,Dd]=tf2ss(N,D);if (isempty(X0));[m,n]=size(A);X0=zeros(1,m); end;
      mask Help: Specify the initial states for the transfer function.  The state ordering is determined by the m-file tf2ss.  There is no unique mapping of the states in a transfer function to states in a state-space representation.  However, tf2ss will consistently use the same mapping for a given transfer function.
      mask Display: dpoly(N,D,'s')
  Transfer Fcn (with initial states)2 : Subsystem  mask(Transfer Function with Initial States){N=[1], D=[600 1], X0=0}
      mask prompts: N "Numerator:"; D "Denominator:"; X0 "Initial conditions:"
      mask help: Vector expressions for numerator, and denominator. Coefficients are in descending powers of s.
      mask init:
      | [A,B,C,Dd]=tf2ss(N,D);if (isempty(X0));[m,n]=size(A);X0=zeros(1,m); end;
      mask Help: Specify the initial states for the transfer function.  The state ordering is determined by the m-file tf2ss.  There is no unique mapping of the states in a transfer function to states in a state-space representation.  However, tf2ss will consistently use the same mapping for a given transfer function.
      mask Display: dpoly(N,D,'s')
  Transfer Fcn (with initial states)3 : Subsystem  mask(Transfer Function with Initial States){N=[1], D=[600 1], X0=0}
      mask prompts: N "Numerator:"; D "Denominator:"; X0 "Initial conditions:"
      mask help: Vector expressions for numerator, and denominator. Coefficients are in descending powers of s.
      mask init:
      | [A,B,C,Dd]=tf2ss(N,D);if (isempty(X0));[m,n]=size(A);X0=zeros(1,m); end;
      mask Help: Specify the initial states for the transfer function.  The state ordering is determined by the m-file tf2ss.  There is no unique mapping of the states in a transfer function to states in a state-space representation.  However, tf2ss will consistently use the same mapping for a given transfer function.
      mask Display: dpoly(N,D,'s')
  on/off ambient : Relay  OnSwitchValue=0.5  OffSwitchValue=-0.5
  on/off hum : Relay  OnSwitchValue=0.5  OffSwitchValue=-0.5
  on/off roomtemp : Relay  OnSwitchValue=0.5  OffSwitchValue=-0.5
  setpoint humidity : Constant  Value=85
  x2RelHum_UIBK : carnot/Basic/Material_Properties/x2RelHum
      settings: SourceProductName=Carnot
  state : Outport  VectorParamsAs1DForOutWhenUnconnected=off
  wires:
  AIB/1 -> Bus Selector5/1
  setpoint/1 -> Sum/1
  Bus Selector5/1 -> Transfer Fcn (with initial states)2/1(In1)  "<Ts>"
  Sum/1 -> on/off roomtemp/1
  on/off roomtemp/1 -> Product/1
  WDB/1 -> Bus Selector1/1
  Bus Selector1/1 -> Transfer Fcn (with initial states)3/1(In1)  "<Temperature_Ambient>"
  Sum1/1 -> on/off ambient/1
  on/off ambient/1 -> Product/2
  Bus Selector5/2 -> x2RelHum_UIBK/1  "<Tc>"
  Bus Selector5/3 -> x2RelHum_UIBK/2  "<p>"
  Bus Selector5/4 -> x2RelHum_UIBK/3  "<x_H2O>"
  Sum2/1 -> on/off hum/1
  x2RelHum_UIBK/1 -> Transfer Fcn (with initial states)1/1(In1)
  setpoint humidity/1 -> Sum2/1
  Add/1 -> Saturation/1
  Product/1 -> Add/2
  on/off hum/1 -> Add/1
  Saturation/1 -> state/1
  Transfer Fcn (with initial states)2/1(Out1) -> Sum1/1, Sum/2
  Transfer Fcn (with initial states)3/1(Out1) -> Sum1/2
  Transfer Fcn (with initial states)1/1(Out1) -> Sum2/2

== system carnotUIBK/HVAC/HVAC_9002_window opening/window opening 6 ==
  setpoint : Inport
  AIB : Inport  Port=2
  WDB : Inport  Port=3
  Enable : EnablePort
  Add : Sum
  Bus Selector1 : BusSelector  OutputSignals=Temperature_Ambient
  Bus Selector5 : BusSelector  OutputSignals=Ts,Tc,p,x_H2O
  Product : Product
  Saturation : Saturate  UpperLimit=1  LowerLimit=0
  Sum : Sum  Inputs=|-+
  Sum1 : Sum  Inputs=|+-
  Sum2 : Sum  Inputs=|-+
  Transfer Fcn (with initial states)1 : Subsystem  mask(Transfer Function with Initial States){N=[1], D=[600 1], X0=0}
      mask prompts: N "Numerator:"; D "Denominator:"; X0 "Initial conditions:"
      mask help: Vector expressions for numerator, and denominator. Coefficients are in descending powers of s.
      mask init:
      | [A,B,C,Dd]=tf2ss(N,D);if (isempty(X0));[m,n]=size(A);X0=zeros(1,m); end;
      mask Help: Specify the initial states for the transfer function.  The state ordering is determined by the m-file tf2ss.  There is no unique mapping of the states in a transfer function to states in a state-space representation.  However, tf2ss will consistently use the same mapping for a given transfer function.
      mask Display: dpoly(N,D,'s')
  Transfer Fcn (with initial states)2 : Subsystem  mask(Transfer Function with Initial States){N=[1], D=[600 1], X0=0}
      mask prompts: N "Numerator:"; D "Denominator:"; X0 "Initial conditions:"
      mask help: Vector expressions for numerator, and denominator. Coefficients are in descending powers of s.
      mask init:
      | [A,B,C,Dd]=tf2ss(N,D);if (isempty(X0));[m,n]=size(A);X0=zeros(1,m); end;
      mask Help: Specify the initial states for the transfer function.  The state ordering is determined by the m-file tf2ss.  There is no unique mapping of the states in a transfer function to states in a state-space representation.  However, tf2ss will consistently use the same mapping for a given transfer function.
      mask Display: dpoly(N,D,'s')
  Transfer Fcn (with initial states)3 : Subsystem  mask(Transfer Function with Initial States){N=[1], D=[600 1], X0=0}
      mask prompts: N "Numerator:"; D "Denominator:"; X0 "Initial conditions:"
      mask help: Vector expressions for numerator, and denominator. Coefficients are in descending powers of s.
      mask init:
      | [A,B,C,Dd]=tf2ss(N,D);if (isempty(X0));[m,n]=size(A);X0=zeros(1,m); end;
      mask Help: Specify the initial states for the transfer function.  The state ordering is determined by the m-file tf2ss.  There is no unique mapping of the states in a transfer function to states in a state-space representation.  However, tf2ss will consistently use the same mapping for a given transfer function.
      mask Display: dpoly(N,D,'s')
  on/off ambient : Relay  OnSwitchValue=0.5  OffSwitchValue=-0.5
  on/off hum : Relay  OnSwitchValue=0.5  OffSwitchValue=-0.5
  on/off roomtemp : Relay  OnSwitchValue=0.5  OffSwitchValue=-0.5
  setpoint humidity : Constant  Value=85
  x2RelHum_UIBK : carnot/Basic/Material_Properties/x2RelHum
      settings: SourceProductName=Carnot
  state : Outport  VectorParamsAs1DForOutWhenUnconnected=off
  wires:
  Transfer Fcn (with initial states)1/1(Out1) -> Sum2/2
  Transfer Fcn (with initial states)3/1(Out1) -> Sum1/2
  Transfer Fcn (with initial states)2/1(Out1) -> Sum/2, Sum1/1
  Saturation/1 -> state/1
  on/off hum/1 -> Add/1
  Product/1 -> Add/2
  Add/1 -> Saturation/1
  setpoint humidity/1 -> Sum2/1
  x2RelHum_UIBK/1 -> Transfer Fcn (with initial states)1/1(In1)
  Sum2/1 -> on/off hum/1
  Bus Selector5/4 -> x2RelHum_UIBK/3  "<x_H2O>"
  Bus Selector5/3 -> x2RelHum_UIBK/2  "<p>"
  Bus Selector5/2 -> x2RelHum_UIBK/1  "<Tc>"
  on/off ambient/1 -> Product/2
  Sum1/1 -> on/off ambient/1
  Bus Selector1/1 -> Transfer Fcn (with initial states)3/1(In1)  "<Temperature_Ambient>"
  WDB/1 -> Bus Selector1/1
  on/off roomtemp/1 -> Product/1
  Sum/1 -> on/off roomtemp/1
  Bus Selector5/1 -> Transfer Fcn (with initial states)2/1(In1)  "<Ts>"
  setpoint/1 -> Sum/1
  AIB/1 -> Bus Selector5/1

== system carnotUIBK/HVAC/HVAC_999_TEMPLATE/Transfer Fcn (with initial states)1 ==
  In1 : Inport
  State Space : StateSpace  A=A  B=B  C=C  D=Dd  InitialCondition=X0
  Out1 : Outport  InitialOutput=0  VectorParamsAs1DForOutWhenUnconnected=off
  wires:
  In1/1 -> State Space/1
  State Space/1 -> Out1/1

== system carnotUIBK/airexchange_intersection/airexchange_empiric/Subsystem ==
  note: (kg/s)
  note: (kg/s)
  note: (kg/s)
  note: (kg/kg)
  note: (kg/kg)
  note: ASSUMPTION: mdot_air_out2in = mdot_air_in2out !
  mdot_air : Inport
  x_in : Inport  Port=2
  x_out : Inport  Port=3
  Demux2 : Demux  Outputs=2
      settings: DisplayOption=none
  Demux3 : Demux  Outputs=2
      settings: DisplayOption=none
  Fcn{,1..3} (4 alike) : Fcn  Expr=u / (1+u)
  Product5 : Product  InputSameDT=on  SaturateOnIntegerOverflow=on  OutDataTypeStr=Inherit: Same as first input
  Product6 : Product  InputSameDT=on  SaturateOnIntegerOverflow=on  OutDataTypeStr=Inherit: Same as first input
  Sum1 : Sum  Inputs=+-  InputSameDT=on  SaturateOnIntegerOverflow=on  OutDataTypeStr=Inherit: Same as first input
  Sum2 : Sum  Inputs=+-  InputSameDT=on  SaturateOnIntegerOverflow=on  OutDataTypeStr=Inherit: Same as first input
  mdot_H2O : Outport  InitialOutput=0  VectorParamsAs1DForOutWhenUnconnected=off
  mdot_CO2 : Outport  Port=2  InitialOutput=0  VectorParamsAs1DForOutWhenUnconnected=off
  wires:
  x_out/1 -> Demux2/1
  Demux2/1 -> Fcn/1  "x_H2O_out"
  Demux2/2 -> Fcn1/1  "x_CO2_out"
  Demux3/2 -> Fcn3/1  "x_CO2_in"
  Demux3/1 -> Fcn2/1  "x_H2O_in"
  x_in/1 -> Demux3/1
  Fcn/1 -> Sum1/1
  Fcn2/1 -> Sum1/2
  Fcn1/1 -> Sum2/1
  Fcn3/1 -> Sum2/2
  Sum2/1 -> Product6/2
  Sum1/1 -> Product5/2
  mdot_air/1 -> Product6/1, Product5/1  "mdot_air >=0"
  Product6/1 -> mdot_CO2/1
  Product5/1 -> mdot_H2O/1

== system carnotUIBK/airexchange_intersection/airexchange_empiric/V exchange ==
  Tc in : Inport
  x in : Inport  Port=2
  Tc out : Inport  Port=3
  x out : Inport  Port=4
  control : Inport  Port=5
  Abs : Abs  SaturateOnIntegerOverflow=off
  Gain1 : Gain  Gain=164.4
  Gain2 : Gain  Gain=32.6/164.4
  Gain4 : Gain  Gain=1000
  Gain5 : Gain  Gain=1000
  Product : Product
  Sum10 : Sum  InputSameDT=on  SaturateOnIntegerOverflow=on  OutDataTypeStr=Inherit: Same as first input
  Sum11 : Sum  Inputs=+-  InputSameDT=on  SaturateOnIntegerOverflow=on  OutDataTypeStr=Inherit: Same as first input
  Sum12 : Sum  Inputs=+-  InputSameDT=on  SaturateOnIntegerOverflow=on  OutDataTypeStr=Inherit: Same as first input
  Sum9 : Sum  InputSameDT=on  SaturateOnIntegerOverflow=on  OutDataTypeStr=Inherit: Same as first input
  "on/off " : Constant  Value=183
  V exchange : Outport  VectorParamsAs1DForOutWhenUnconnected=off
  wires:
  Sum12/1 -> Gain2/1
  Gain1/1 -> Sum10/2
  Abs/1 -> Gain1/1
  Sum9/1 -> Abs/1
  Gain2/1 -> Sum9/2
  "on/off "/1 -> Sum10/1
  Sum11/1 -> Sum9/1
  Tc out/1 -> Sum11/2
  x in/1 -> Gain4/1
  Tc in/1 -> Sum11/1
  x out/1 -> Gain5/1
  Sum10/1 -> Product/1
  Product/1 -> V exchange/1
  Gain4/1 -> Sum12/1
  Gain5/1 -> Sum12/2
  control/1 -> Product/2

== system carnotUIBK/airexchange_intersection/airexchange_powerlaw/Subsystem ==
  note: (kg/s)
  note: (kg/s)
  note: (kg/s)
  note: (kg/kg)
  note: (kg/kg)
  note: ASSUMPTION: mdot_air_out2in = mdot_air_in2out !
  mdot_air : Inport
  x_in : Inport  Port=2
  x_out : Inport  Port=3
  Demux2 : Demux  Outputs=2
      settings: DisplayOption=none
  Demux3 : Demux  Outputs=2
      settings: DisplayOption=none
  Fcn{,1..3} (4 alike) : Fcn  Expr=u / (1+u)
  Product5 : Product  InputSameDT=on  SaturateOnIntegerOverflow=on  OutDataTypeStr=Inherit: Same as first input
  Product6 : Product  InputSameDT=on  SaturateOnIntegerOverflow=on  OutDataTypeStr=Inherit: Same as first input
  Sum1 : Sum  Inputs=+-  InputSameDT=on  SaturateOnIntegerOverflow=on  OutDataTypeStr=Inherit: Same as first input
  Sum2 : Sum  Inputs=+-  InputSameDT=on  SaturateOnIntegerOverflow=on  OutDataTypeStr=Inherit: Same as first input
  mdot_H2O : Outport  InitialOutput=0  VectorParamsAs1DForOutWhenUnconnected=off
  mdot_CO2 : Outport  Port=2  InitialOutput=0  VectorParamsAs1DForOutWhenUnconnected=off
  wires:
  x_out/1 -> Demux2/1
  Demux2/1 -> Fcn/1  "x_H2O_out"
  Demux2/2 -> Fcn1/1  "x_CO2_out"
  Demux3/2 -> Fcn3/1  "x_CO2_in"
  Demux3/1 -> Fcn2/1  "x_H2O_in"
  x_in/1 -> Demux3/1
  Fcn/1 -> Sum1/1
  Fcn2/1 -> Sum1/2
  Fcn1/1 -> Sum2/1
  Fcn3/1 -> Sum2/2
  Sum2/1 -> Product6/2
  Sum1/1 -> Product5/2
  mdot_air/1 -> Product6/1, Product5/1  "mdot_air >=0"
  Product6/1 -> mdot_CO2/1
  Product5/1 -> mdot_H2O/1

== system carnotUIBK/airexchange_intersection/airexchange_powerlaw/door open ==
  H (height of the door [m]) : Inport
  rho_i : Inport  Port=2
  rho_j : Inport  Port=3
  L : Inport  Port=4
  control : Inport  Port=5
  Abs : Abs  SaturateOnIntegerOverflow=off
  Abs1 : Abs  SaturateOnIntegerOverflow=off
  Abs2 : Abs  SaturateOnIntegerOverflow=off
  Add : Sum
  Cd : Constant  Value=0.78
  Constant1 : Constant  Value=0.5
  Constant2 : Constant  Value=0.5
  Constant3 : Constant  Value=0.5
  Math Function : Math  Operator=pow  SignedPower=on
  Math Function1 : Math  Operator=pow  SignedPower=on
  Product : Product
  Product2 : Product  Inputs=3
  Product3 : Product
  Product6 : Product  Inputs=5
  d_rho : Sum  Inputs=+-
  g : Constant  Value=9.81
  mean : Gain  Gain=0.5
  sqrt(2)/2 : Gain  Gain=0.707106781
  m_dot_open_door : Outport  VectorParamsAs1DForOutWhenUnconnected=off
  wires:
  Product3/1 -> Product/2
  control/1 -> Product/1
  Product/1 -> m_dot_open_door/1
  d_rho/1 -> Product2/3
  Product2/1 -> Abs/1
  g/1 -> Product2/2
  Math Function/1 -> Product3/2
  Constant2/1 -> Math Function/2
  Abs/1 -> Math Function/1
  Product6/1 -> Abs2/1  "C_coeff"
  mean/1 -> Abs1/1
  sqrt(2)/2/1 -> Product6/1
  Add/1 -> mean/1
  H (height of the door [m])/1 -> Product2/1, Product6/3
  rho_j/1 -> Add/2, d_rho/2
  rho_i/1 -> d_rho/1, Add/1
  L/1 -> Product6/2
  Cd/1 -> sqrt(2)/2/1
  Constant1/1 -> Product6/5
  Constant3/1 -> Math Function1/2
  Abs1/1 -> Math Function1/1
  Math Function1/1 -> Product6/4
  Abs2/1 -> Product3/1

== system carnotUIBK/gain/Equipment/W//device ==
  Switch : Inport
  Constant13 : Constant  Value=zeros(1,14)
  Constant14 : Constant  Value=zeros(1,2)
  Gain1 : Gain  Gain=0.6  SaturateOnIntegerOverflow=on  OutDataTypeStr=Inherit: Same as input  ParamDataTypeStr=Inherit: Same as input
  Gain4 : Gain  Gain=0.4  SaturateOnIntegerOverflow=on  OutDataTypeStr=Inherit: Same as input  ParamDataTypeStr=Inherit: Same as input
  Mux1 : Mux  Inputs=[1 1 14 1 2]
  Product1 : Product
  Profile W/device : carnot/Load/General/Repeating_Profile  period=timevalues(end)  rep_seq_t=timevalues(1:end-1)  rep_seq_d=timeduration  rep_seq_y=values1
      settings: SourceProductName=Carnot
  timeconstant : simulink_extras/Additional Linear/Transfer Fcn (with initial outputs)  N=[1]  D=[60 1]  Y0=0  U0=0
  "[S]" : Outport  VectorParamsAs1DForOutWhenUnconnected=off
  wires:
  Product1/1 -> "[S]"/1
  Switch/1 -> Product1/1
  Gain4/1 -> Mux1/2
  Mux1/1 -> Product1/2
  Gain1/1 -> Mux1/1
  Profile W/device/1 -> timeconstant/1
  Constant13/1 -> Mux1/3
  Constant14/1 -> Mux1/5
  timeconstant/1 -> Mux1/4, Gain4/1, Gain1/1

== system carnotUIBK/gain/Equipment/W//m² ==
  Switch : Inport
  Constant1 : Constant  Value=zeros(1,14)
  Constant2 : Constant  Value=zeros(1,2)
  Gain1 : Gain  Gain=z.heated_area  SaturateOnIntegerOverflow=on  OutDataTypeStr=Inherit: Same as input  ParamDataTypeStr=Inherit: Same as input
  Gain3 : Gain  Gain=0.6  SaturateOnIntegerOverflow=on  OutDataTypeStr=Inherit: Same as input  ParamDataTypeStr=Inherit: Same as input
  Gain5 : Gain  Gain=0.4  SaturateOnIntegerOverflow=on  OutDataTypeStr=Inherit: Same as input  ParamDataTypeStr=Inherit: Same as input
  Mux2 : Mux  Inputs=[1 1 14 1 2]
  Product : Product
  Profile W/m² : carnot/Load/General/Repeating_Profile  period=timevalues(end)  rep_seq_t=timevalues(1:end-1)  rep_seq_d=timeduration  rep_seq_y=values1
      settings: SourceProductName=Carnot
  timeconstant : simulink_extras/Additional Linear/Transfer Fcn (with initial outputs)  N=[1]  D=[60 1]  Y0=0  U0=0
  "[S]" : Outport  VectorParamsAs1DForOutWhenUnconnected=off
  wires:
  Product/1 -> "[S]"/1
  Switch/1 -> Product/1
  Gain5/1 -> Mux2/2
  Mux2/1 -> Product/2
  Gain3/1 -> Mux2/1
  Profile W/m²/1 -> Gain1/1
  Gain1/1 -> timeconstant/1
  Constant1/1 -> Mux2/3
  Constant2/1 -> Mux2/5
  timeconstant/1 -> Mux2/4, Gain5/1, Gain3/1
